simulink subsystem "SPWM_modulator_VSI"  (R2022b)
settings: Solver=VariableStepAuto  StartTime=0.0  StopTime=10.0  RelTol=1e-3
libraries: spsTriangleGeneratorLib x1
settings Model: Creator=jack  LastModifiedBy=jack

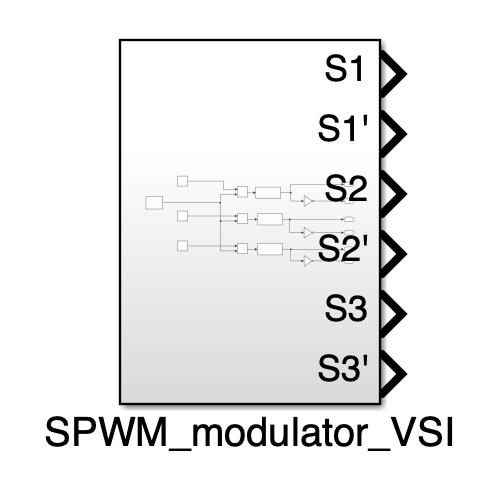
[thumbnail: Simulink's stored preview of the top-level diagram]
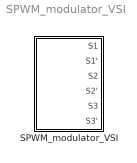
== system SPWM_modulator_VSI ==
  SPWM_modulator_VSI : Subsystem

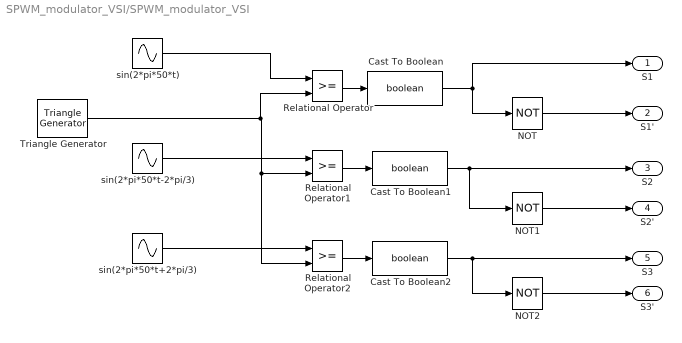
== system SPWM_modulator_VSI/SPWM_modulator_VSI ==
  Cast To Boolean : DataTypeConversion  OutDataTypeStr=boolean  SaturateOnIntegerOverflow=off  RndMeth=Floor
  Cast To Boolean1 : DataTypeConversion  OutDataTypeStr=boolean  SaturateOnIntegerOverflow=off  RndMeth=Floor
  Cast To Boolean2 : DataTypeConversion  OutDataTypeStr=boolean  SaturateOnIntegerOverflow=off  RndMeth=Floor
  NOT : Logic  Operator=NOT  IconShape=distinctive  AllPortsSameDT=off  OutDataTypeStr=boolean
  NOT1 : Logic  Operator=NOT  IconShape=distinctive  AllPortsSameDT=off  OutDataTypeStr=boolean
  NOT2 : Logic  Operator=NOT  IconShape=distinctive  AllPortsSameDT=off  OutDataTypeStr=boolean
  Relational Operator : RelationalOperator  OutDataTypeStr=boolean  RndMeth=Simplest  InputSameDT=off
  Relational Operator1 : RelationalOperator  OutDataTypeStr=boolean  RndMeth=Simplest  InputSameDT=off
  Relational Operator2 : RelationalOperator  OutDataTypeStr=boolean  RndMeth=Simplest  InputSameDT=off
  Triangle Generator : spsTriangleGeneratorLib/Triangle Generator  Freq=2e3  Phase=90  Ts=0
  sin(2*pi*50*t) : Sin  Frequency=2*pi*50  SampleTime=0
  sin(2*pi*50*t+2*pi/3) : Sin  Frequency=2*pi*50  Phase=2*pi/3  SampleTime=0
  sin(2*pi*50*t-2*pi/3) : Sin  Frequency=2*pi*50  Phase=-2*pi/3  SampleTime=0
  S1 : Outport
  S1' : Outport  Port=2
  S2 : Outport  Port=3
  S2' : Outport  Port=4
  S3 : Outport  Port=5
  S3' : Outport  Port=6
  wires:
  NOT1/1 -> S2'/1
  Relational Operator1/1 -> Cast To Boolean1/1
  sin(2*pi*50*t+2*pi/3)/1 -> Relational Operator2/1
  Relational Operator/1 -> Cast To Boolean/1
  sin(2*pi*50*t-2*pi/3)/1 -> Relational Operator1/1
  Cast To Boolean/1 -> S1/1, NOT/1
  Relational Operator2/1 -> Cast To Boolean2/1
  Cast To Boolean1/1 -> S2/1, NOT1/1
  Cast To Boolean2/1 -> S3/1, NOT2/1
  Triangle Generator/1 -> Relational Operator/2, Relational Operator2/2, Relational Operator1/2
  NOT/1 -> S1'/1
  NOT2/1 -> S3'/1
  sin(2*pi*50*t)/1 -> Relational Operator/1
